simulink model "State_Feedback_Linear"  (R2022b)
settings: Solver=FixedStepAuto  StartTime=0.0  StopTime=15  FixedStep=step_size  RelTol=1e-3
undefined symbols (not defined in the file): a, theta_i, x_i, y_i, zeta
libraries: simulink_extras x2
settings Model: PauseTimes=14.13  Creator=Musta  LastModifiedBy=Musta

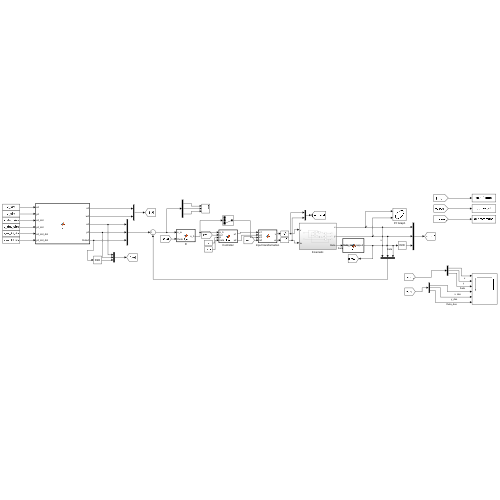
[thumbnail: Simulink's stored preview of the top-level diagram]
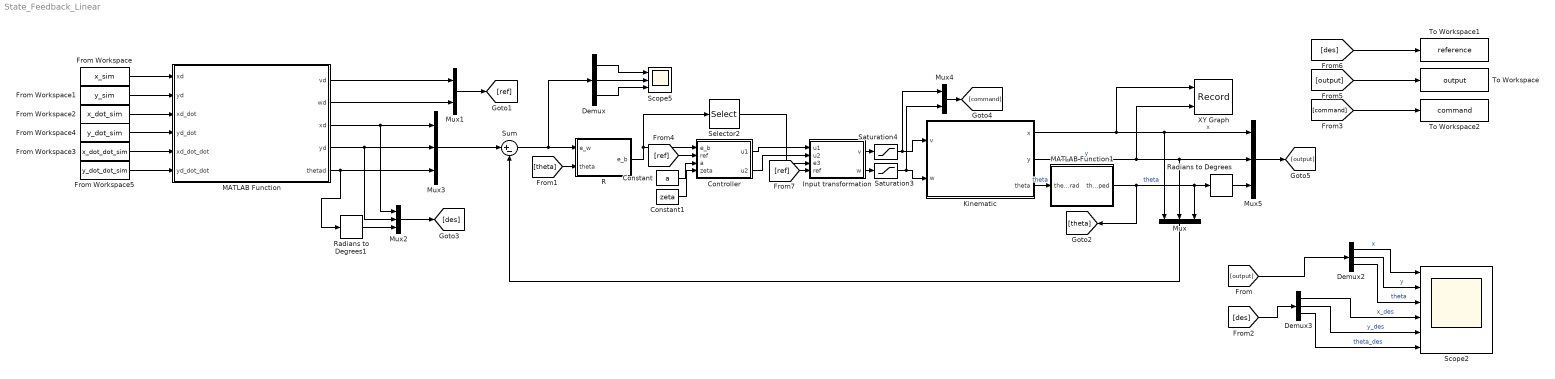
== system State_Feedback_Linear ==
  Constant : Constant  Value=a
  Constant1 : Constant  Value=zeta
  Controller : MATLAB Function  TreatAsAtomicUnit=on
  Demux : Demux  Outputs=3
  Demux2 : Demux  Outputs=3
  Demux3 : Demux  Outputs=3
  From Workspace : FromWorkspace  VariableName=x_sim
  From Workspace1 : FromWorkspace  VariableName=y_sim
  From Workspace2 : FromWorkspace  VariableName=x_dot_sim
  From Workspace3 : FromWorkspace  VariableName=x_dot_dot_sim
  From Workspace4 : FromWorkspace  VariableName=y_dot_sim
  From Workspace5 : FromWorkspace  VariableName=y_dot_dot_sim
  Input transformation : MATLAB Function  TreatAsAtomicUnit=on
  Kinematic : Subsystem
  MATLAB Function : MATLAB Function  TreatAsAtomicUnit=on
  MATLAB Function1 : MATLAB Function  TreatAsAtomicUnit=on
  Mux{,2..3,5} (4 alike) : Mux  Inputs=3
  Mux1 : Mux  Inputs=2
  Mux4 : Mux  Inputs=2
  R : MATLAB Function  TreatAsAtomicUnit=on
  Radians to Degrees : simulink_extras/Transformations/Radians to Degrees
  Radians to Degrees1 : simulink_extras/Transformations/Radians to Degrees
  Saturation3 : Saturate  UpperLimit=2  LowerLimit=-2
  Saturation4 : Saturate  UpperLimit=2  LowerLimit=-2
  Scope2 : Scope  NumInputPorts=6
  Scope5 : Scope  NumInputPorts=3
  Selector2 : Selector  InputPortWidth=3  IndexOptions=Index vector (dialog)  Indices=3  OutputSizes=1
  Sum : Sum  Inputs=|+-
  To Workspace : ToWorkspace  VariableName=output  SaveFormat=Structure With Time  SampleTime=-1
  To Workspace1 : ToWorkspace  VariableName=reference  SaveFormat=Structure With Time  SampleTime=-1
  To Workspace2 : ToWorkspace  VariableName=command  SaveFormat=Structure With Time  SampleTime=-1
  XY Graph : Record  FileSettingsInternal="{\"entries\":[{\"content\":{\"excelSettings\":{\"content\":{},\"type\":\"Streamout.ExcelSettings\"}},\"type\":\"Streamout.FileSettingStorage\",\"uuid\":\"127064ea-453b-4edf-8e8f-cb0125d091b6\"}],\"packageUris\":[\"http://schema.mathworks.com/mf0/streamout_blocks/R2020a\"],\"version\":\"1.0\"}"  Layout=[1 1]  SignalsInternal="{\"entries\":[{\"content\":{\"signals\":[{\"content\":{\"blockPath\":[\"State_Feedback_Linear/XY Graph\"],\"channel\":[],\"dimensions\":[1],\"domain\":\"State_Feedback_Linear/XY Graph\",\"lineColor\":\"#0072bd\",\"plots\":[],\"port\":1,\"sid\":[\"\"],\"signalID\":250,\"signalName\":\"x\"},\"type\":\"RecordBlkView.Signal\",\"uuid\":\"4291d05a-3eea-4163-9088-bf1ae68c7bc7\"},{\"content\":{\"blockPath\":[\"State_Feedback_Linear/XY Graph\"],\"channel\":[],\"dimensions\":[1],\"domain\":\"State_Feedback_Linear/XY Graph\",\"lineColor\":\"#d95319\",\"plots\":[],\"port\":2,\"sid\":[\"\"],\"signalID\":254,\"signalName\":\"y\"},\"type\":\"RecordBlkView.Signal\",\"uuid\":\"27da98a3-47bd-4fba-84d7-d513c880ca6a\"}]},\"type\":\"RecordBlkView.InputSignals\",\"uuid\":\"854b996e-2a02-4fd1-9805-2f599cbdc4fb\"}],\"packageUris\":[\"http://schema.mathworks.com/mf0/streamout_blocks/R2020a\"],\"version\":\"1.0\"}"  VisualizationBindings="{\"xyplotplugin\":{\"info\":[{\"series\":[],\"subplotID\":1}]}}"  CompatibilityTag=XY
  wires:
  Demux3/2 -> Scope2/5  "y_des"
  Mux3/1 -> Sum/1
  Demux2/2 -> Scope2/2  "y"
  [des] -> To Workspace1/1
  [output] -> Demux2/1
  Demux3/1 -> Scope2/4  "x_des"
  [output] -> To Workspace/1
  Mux2/1 -> [des]
  [des] -> Demux3/1
  Demux2/3 -> Scope2/3  "theta"
  Sum/1 -> R/1(e_w), Demux/1
  Demux2/1 -> Scope2/1  "x"
  MATLAB Function/5(thetad) -> Mux3/3, Radians to Degrees1/1
  [theta] -> R/2(theta)
  R/1(e_b) -> Selector2/1, Controller/1(e_b)
  Controller/1(u1) -> Input transformation/1(u1)
  [ref] -> Controller/2(ref)
  Input transformation/2(w) -> Saturation3/1
  Controller/2(u2) -> Input transformation/2(u2)
  [ref] -> Input transformation/4(ref)
  Selector2/1 -> Input transformation/3(e3)
  Kinematic/3(theta) -> MATLAB Function1/1(theta_rad)  "theta"
  Constant/1 -> Controller/3(a)
  Constant1/1 -> Controller/4(zeta)
  Demux3/3 -> Scope2/6  "theta_des"
  Demux/1 -> Scope5/1
  Demux/2 -> Scope5/2
  Demux/3 -> Scope5/3
  From Workspace2/1 -> MATLAB Function/3(xd_dot)
  From Workspace4/1 -> MATLAB Function/4(yd_dot)
  MATLAB Function/2(wd) -> Mux1/2
  MATLAB Function/1(vd) -> Mux1/1
  MATLAB Function/3(xd) -> Mux2/1, Mux3/1
  MATLAB Function/4(yd) -> Mux2/2, Mux3/2
  From Workspace/1 -> MATLAB Function/1("xd ")
  From Workspace1/1 -> MATLAB Function/2("yd ")
  From Workspace5/1 -> MATLAB Function/6(yd_dot_dot)
  From Workspace3/1 -> MATLAB Function/5(xd_dot_dot)
  Mux1/1 -> [ref]
  [command] -> To Workspace2/1
  Saturation3/1 -> Mux4/2, Kinematic/2(w)
  Mux4/1 -> [command]
  Saturation4/1 -> Mux4/1, Kinematic/1(v)
  Input transformation/1(v) -> Saturation4/1
  Mux5/1 -> [output]
  MATLAB Function1/1(theta_rad_wrapped) -> Mux/3, Radians to Degrees/1, [theta]  "theta"
  Radians to Degrees/1 -> Mux5/3
  Mux/1 -> Sum/2
  Kinematic/2(y) -> XY Graph/2, Mux/2, Mux5/2  "y"
  Kinematic/1(x) -> XY Graph/1, Mux/1, Mux5/1  "x"
  Radians to Degrees1/1 -> Mux2/3

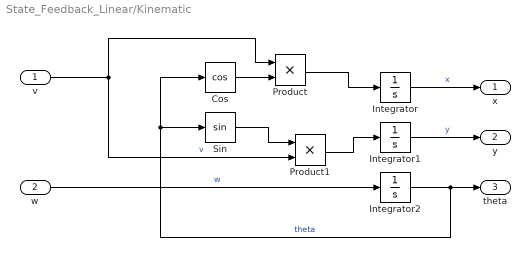
== system State_Feedback_Linear/Kinematic ==
  v : Inport
  w : Inport  Port=2
  Cos : Trigonometry  Operator=cos
  Integrator : Integrator  InitialCondition=x_i
  Integrator1 : Integrator  InitialCondition=y_i
  Integrator2 : Integrator  InitialCondition=theta_i
  Product : Product
  Product1 : Product
  Sin : Trigonometry
  x : Outport
  y : Outport  Port=2
  theta : Outport  Port=3
  wires:
  w/1 -> Integrator2/1  "w"
  Product/1 -> Integrator/1
  v/1 -> Product/1, Product1/2  "v"
  Cos/1 -> Product/2
  Integrator1/1 -> y/1  "y"
  Integrator/1 -> x/1  "x"
  Integrator2/1 -> Cos/1, Sin/1, theta/1  "theta"
  Product1/1 -> Integrator1/1
  Sin/1 -> Product1/1

== matlab function State_Feedback_Linear/R ==
  data: e_w input; e_b output; theta input
function e_b  = fcn(e_w, theta)
    
    R = [cos(theta), sin(theta), 0;
        -sin(theta), cos(theta), 0;
         0, 0, 1];

    e_b = R * e_w;

end

== matlab function State_Feedback_Linear/MATLAB Function ==
  data: xd input; vd output; yd input; xd_dot input; yd_dot input; xd_dot_dot input; yd_dot_dot input; wd output; xd output; yd output; thetad output
function [vd, wd, xd, yd, thetad] = fcn(xd, yd, xd_dot, yd_dot, xd_dot_dot, yd_dot_dot)
    
    vd = sqrt(xd_dot.^2 + yd_dot.^2);
    wd = (xd_dot.*yd_dot_dot - xd_dot_dot.*yd_dot) / (xd_dot.^2 + yd_dot.^2);
    % thetad = atan2(yd_dot, xd_dot);
    thetad = mod(atan2(yd_dot,xd_dot), 2*pi);

    xd = xd;
    yd = yd;

end

== matlab function State_Feedback_Linear/Controller ==
  data: e_b input; u1 output; ref input; u2 output; a input; zeta input
function [u1,u2] = fcn(e_b, ref, a, zeta)

    k1 = 2*zeta*a;
    k2 = (a^2 - ref(2)^2) / ref(1);
    k3 = 2*zeta*a;

    u1 = -k1*e_b(1);
    u2 = -k2*e_b(2) -k3*e_b(3);

end

== matlab function State_Feedback_Linear/Input transformation ==
  data: u1 input; v output; u2 input; e3 input; w output; ref input
function [v, w] = fcn(u1, u2, e3, ref)

    v = ref(1)*cos(e3) - u1;
    w = ref(2) - u2;

end

== matlab function State_Feedback_Linear/MATLAB Function1 ==
  data: theta_rad input; theta_rad_wrapped output
function theta_rad_wrapped = fcn(theta_rad)

    if abs(theta_rad) < 5e-5
        theta_rad = 0;
    end

    theta_rad_wrapped = wrapTo2Pi(theta_rad);

end
